simulink model "matlabFcnTest"  (R2021a)
settings: Solver=ode4  StartTime=0.0  StopTime=10.0  FixedStep=0.001  RelTol=1e-3
settings Model: Creator=jadg1  LastModifiedBy=jadg1

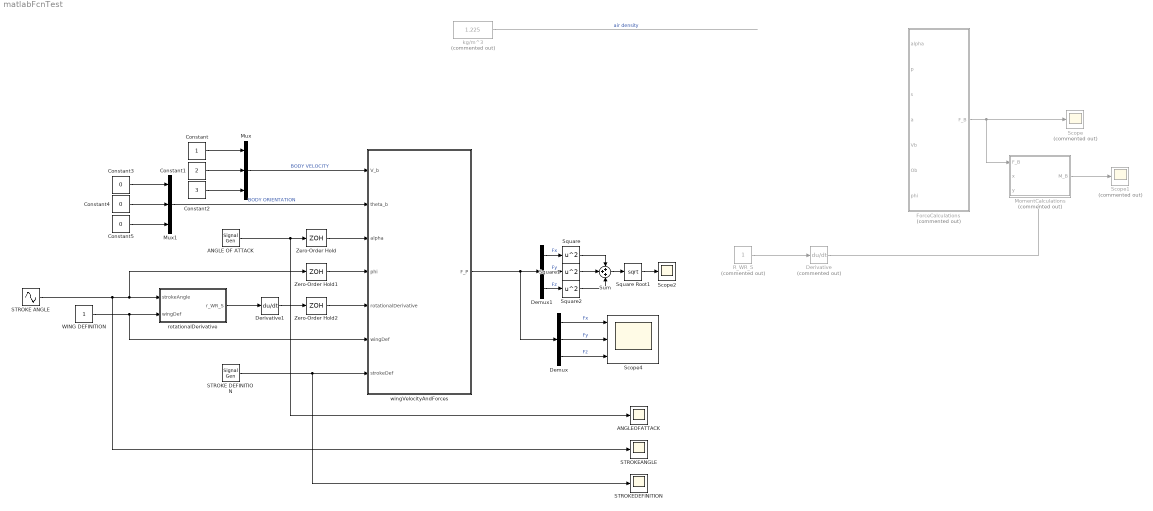
== system matlabFcnTest ==
  ANGLE OF ATTACK : SignalGenerator  WaveForm=square  Amplitude=pi()/6  Frequency=50  Units=rad/sec
  ANGLEOFATTACK : Scope
  Constant : Constant
  Constant1 : Constant  Value=2
  Constant2 : Constant  Value=3
  Constant3 : Constant  Value=0
  Constant4 : Constant  Value=0
  Constant5 : Constant  Value=0
  Demux : Demux  Outputs=3
  Demux1 : Demux  Outputs=3
  Derivative : Derivative  Commented=on
  Derivative1 : Derivative
  ForceCalculations : MATLAB Function  Commented=on  TreatAsAtomicUnit=on
  MomentCalculations : MATLAB Function  Commented=on  TreatAsAtomicUnit=on
  Mux : Mux  Inputs=3
  Mux1 : Mux  Inputs=3
  R_WR_S : Constant  Commented=on
  STROKE ANGLE : Sin  Amplitude=pi()/2  Frequency=50  Phase=pi()/2  SampleTime=0
  STROKE DEFINITION : SignalGenerator  WaveForm=square  Frequency=50  Units=rad/sec
  STROKEANGLE : Scope
  STROKEDEFINITION : Scope
  Scope : Scope  Commented=on
  Scope1 : Scope  Commented=on
  Scope2 : Scope
  Scope4 : Scope  NumInputPorts=3
  Square : Math  Operator=square  SaturateOnIntegerOverflow=on
  Square Root1 : Sqrt  SaturateOnIntegerOverflow=on
  Square1 : Math  Operator=square  SaturateOnIntegerOverflow=on
  Square2 : Math  Operator=square  SaturateOnIntegerOverflow=on
  Sum : Sum  Inputs=+++
  WING DEFINITION : Constant
  Zero-Order Hold : ZeroOrderHold  SampleTime=-1
  Zero-Order Hold1 : ZeroOrderHold  SampleTime=-1
  Zero-Order Hold2 : ZeroOrderHold  SampleTime=-1
  kg/m^3 : Constant  Commented=on  Value=1.225
  rotationalDerivative : MATLAB Function  TreatAsAtomicUnit=on
  wingVelocityAndForces : MATLAB Function  TreatAsAtomicUnit=on
  wires:
  ForceCalculations/1(F_B) -> Scope/1, MomentCalculations/1(F_B)
  MomentCalculations/1(M_B) -> Scope1/1
  Constant/1 -> Mux/1
  Constant1/1 -> Mux/2
  Constant2/1 -> Mux/3
  Constant5/1 -> Mux1/3
  Constant4/1 -> Mux1/2
  Constant3/1 -> Mux1/1
  Mux/1 -> wingVelocityAndForces/1(V_b)  "BODY VELOCITY"
  STROKE DEFINITION/1 -> STROKEDEFINITION/1, wingVelocityAndForces/7(strokeDef)
  ? -> ForceCalculations/1(alpha)
  ? -> ForceCalculations/2(p)
  ? -> ForceCalculations/3(s)
  ? -> ForceCalculations/4(a)
  ? -> ForceCalculations/5(Vb)
  ? -> ForceCalculations/6(Ob)
  ? -> ForceCalculations/7(phi)
  kg/m^3/1 -> ?  "air density"
  Mux1/1 -> wingVelocityAndForces/2(theta_b)  "BODY ORIENTATION"
  Derivative/1 -> ?
  R_WR_S/1 -> Derivative/1
  ANGLE OF ATTACK/1 -> ANGLEOFATTACK/1, Zero-Order Hold/1
  STROKE ANGLE/1 -> STROKEANGLE/1, Zero-Order Hold1/1, rotationalDerivative/1(strokeAngle)
  WING DEFINITION/1 -> wingVelocityAndForces/6(wingDef), rotationalDerivative/2(wingDef)
  rotationalDerivative/1(r_WR_S) -> Derivative1/1
  Derivative1/1 -> Zero-Order Hold2/1
  wingVelocityAndForces/1(F_P) -> Demux1/1, Demux/1
  Zero-Order Hold/1 -> wingVelocityAndForces/3(alpha)
  Zero-Order Hold1/1 -> wingVelocityAndForces/4(phi)
  Zero-Order Hold2/1 -> wingVelocityAndForces/5(rotationalDerivative)
  Demux/1 -> Scope4/1  "Fx"
  Demux/2 -> Scope4/2  "Fy"
  Demux/3 -> Scope4/3  "Fz"
  Sum/1 -> Square Root1/1
  Demux1/1 -> Square/1  "Fx"
  Square Root1/1 -> Scope2/1
  Demux1/2 -> Square1/1  "Fy"
  Demux1/3 -> Square2/1  "Fz"
  Square/1 -> Sum/1
  Square1/1 -> Sum/2
  Square2/1 -> Sum/3

== matlab function matlabFcnTest/MomentCalculations ==
  data: F_B input; x input; y input; M_B output
function M_B = testFcn(F_B,x,y)

M_B = F_B^2 * y^2;

end

== matlab function matlabFcnTest/ForceCalculations ==
  data: alpha input; F_B output; p input; s input; a input; Vb input; Ob input; phi input
function F_B = testFcn(alpha,p,s,a,Vb,Ob,phi)

wingVelocity = [1;2;3];

liftCoeff = 1.58*sin((2.13*alpha)-(7.2*(pi()/180))) + 0.225;

dragCoeff = 1.92 - 1.55*cos((2.04*alpha)-(9.82*(pi()/180)));

densityCoeff = p/2;

dL_V = densityCoeff * norm(wingVelocity)*liftCoeff;

dD_V = densityCoeff * norm(wingVelocity)*dragCoeff;

dF_V = [ sign(alpha)*dl_V ; dD_V ; 0 ];

% Creating the rotation matrix R_V_P



% ROTATE TO BECOME dF_P

%{ 
WHAT WE NEED TO END WITH

F_P = integral2(dF_P,0,c,0,r)

%}

a = 1;

F_B = testFunction3(a,dL_V,dD_V);


function output = testFunction3(a,x,y)

output = x.*y + a;

end



%{
F_B_1 = alpha*p*s*a*phi;

F_B_2 = F_B_1*Vb;

F_B = F_B_2*Ob;
%}




end

== matlab function matlabFcnTest/wingVelocityAndForces ==
  data: V_b input; theta_b input; alpha input; phi input; rotationalDerivative input; wingDef input; strokeDef input; F_P output
function F_P = WingVelocityAndForces(V_b, theta_b, alpha, phi, rotationalDerivative, wingDef, strokeDef)
% DESCRIPTION:
% This function is required to use symbolic variables by defining every
% function called as an extrinsic function.

% Define each function as an extrinsic function:
coder.extrinsic('wingForces');
coder.extrinsic('wingVelocity');

% Define the output size:
F_P = zeros(3,1);

% Call the function that calculates the wing velocity and forces
F_P = wingForces(V_b, theta_b, alpha, phi, rotationalDerivative, wingDef, strokeDef);

%{
    % Calculation of the wing force
    function wingForce = wingForces(V_b, theta_b, alpha, phi, rotationalDerivative, wingDef, strokeDef)

    % THIS LINE OF CODE IS TEMPORARY AND MUST BE REMOVED
    psi = pi()/4;


    % Define the r and c values:

    syms r;
    syms c;

    r_max = 2;
    c_max = 1;


    % Calculate the coefficients:

    densityCoeff = 1.225/2;

    liftCoeff = 1.58*sin((2.13*alpha)-(7.2*(pi()/180))) + 0.225;

    dragCoeff = 1.92 - 1.55*cos((2.04*alpha)-(9.82*(pi()/180)));


    % Calculate the magnitude of the wing velocity:

    wingVelocity_P = wingVelocity(V_b, theta_b, alpha, phi, rotationalDerivative, wingDef, strokeDef);

    wingVelocityMagnitude = norm(wingVelocity_P);


    % Calculate the infinitesimal lift and drag:

    dL_V = densityCoeff * wingVelocityMagnitude * liftCoeff;

    dD_V = densityCoeff * wingVelocityMagnitude * dragCoeff;


    % Construct the force vector:

    dF_V = [ sign(alpha)*dL_V ; dD_V ; 0 ];

    % Generate the rotational matrix from the V to the P frame:

    r_PP_V = R_PP_V(alpha);
    r_V_PP = r_PP_V^(-1);

    r_P_PP = R_P_PP(psi);
    r_PP_P = r_P_PP^(-1);

    r_V_P = r_V_PP * r_PP_P;

    % Transform the force vector to the correct frame:

    coder.extrinsic('vpa');

    dF_P = vpa(r_V_P * dF_V);

    wingForce = double(int(int(dF_P,c,-c_max,0),0,r_max));
    
    end


    % Calculation of the wing velocity
    function wingVelocity = wingVelocity(V_b, theta_b, alpha, phi, rotationalDerivative, wingDef, strokeDef)

    % Definitions: B-Body Frame; S-Spar Frame; P- Planform Frame; wr- Wing Root; ws-Wing Spar;
    % wp-Wing planform; 

    % Distance from the centre of gravity to the base of the wing root
    r_CG_WR = [0;1;2];              

    % Rotation matrix of the rigid body from inertial frame the body frame
    r_I_B = R_I_B(theta_b);

    % Rotation matrix from the spar frame to the planform frame
    r_S_P = R_S_P(strokeDef, alpha);

    % Rotation matrix from the wing root frame to the spar frame
    r_WR_S = R_WR_S(wingDef, phi);

    % rotation of body frame in spar frame coordinates
    R_B_S = r_WR_S *  r_S_P; 

    % Using the upstroke, left wing definition
    %{
    % Wing movements definition 

    u= 1;    % upstroke 
    d = -1;  % downstroke 

    % left wing and right wing definition
    wingDef = 1;             % Left wing
    %s = -1;            % Right wing
    %}

    % Position vector of infinitesimal point on body frame(r_B); spar frame (r_S), and planform (r_P)
    syms r c;
    r_P = [0; r; -c];                           % Position vector of infinitesimal point on wing planform (r_P)
    r_B = (r_CG_WR)+ r_WR_S * r_S_P * r_P;   % Position vector of infinitesimal point on rigid body (r_B)
    r_S = r_S_P * r_P;                          % Position vector of infinitesimal point on spar frame (r_S)

    % Velocity due to rigid body rotation

    Wb_B = transpose(r_I_B);                % angular velocity of body frame with respect to changng theta with time                   % 
    V_r =  r_WR_S * Wb_B * r_B;           % FINAL 1

    %{
    if s == 1 && u == 1 
    V_r = r_WR_S  * u * Wb_B * r_B;  % left wing upstroke
    end 


    if s == 1 && d == -1 
    V_r = r_WR_S * d * Wb_B * r_B;  % left wing downstroke
    end 
    %}
    if wingDef == -1 && d == -1
    V_r = r_WR_S * d * Wb_B * r_B;  % right wing downstroke 
    end 

    %{
    if s == -1 && u == 1
    V_r = r_WR_S * u * Wb_B * r_B;  % right wing upstroke 
    end 
    %}

    % Velocity due to rigid body translation

    % position vector for centre of gravity of rigid body to wing root on body frame

     V_b_B = V_b + (Wb_B * r_CG_WR);       % evaluation of rigid body velocity of body frame

     V_t = R_B_S * V_b_B;                % FINAL 2

    %Velocity due to wing flapping

    V_f = r_WR_S * rotationalDerivative * r_S;                   % FINAL 3

    wingVelocity = vpa(V_r + V_t + V_f);                % Free stream velocity over an incremental area of wing planform (Addition of FINAL 1 to FINAL 3) 

    end
%}

end

== matlab function matlabFcnTest/rotationalDerivative ==
  data: strokeAngle input; wingDef input; r_WR_S output
function r_WR_S = R_WR_S(strokeAngle,wingDef)

%R_WR_S Return rotation matrix for wing root frame to wing spar frame
%   wingDef = wing parameter
%       s = 1 left wing
%       s = -1 right wing
%   strokeAngle = stroke angle (rad) 

% left/right wing correction angle
x = -(1-wingDef)*pi/2;

% convert radians to degrees
phi = rad2deg(strokeAngle);
x = rad2deg(x); % 

% Rotate about z-axis
r_WR_S = rotz(x + wingDef*strokeAngle);

end
